simulink model "fxio_i2c_slave_rx_s32k11x"  (Simulink 9.0)
settings: Solver=FixedStepDiscrete  StartTime=0.0  StopTime=10.0  FixedStep=0.1  RelTol=1e-3
InitFcn:
  | mbd_s32k_consistency_checks(bdroot(gcs));
undefined symbols (not defined in the file): LQFP, thumb
libraries: mbd_s32k1xx_ec_toolbox x6, simulink x1
Description:
  | I2C Slave - to be used for FlexIO Master examples.
  | Note: FlexIO is limited to Master-only emulation for I2C - so LPI2C instance must be used for the Slave.
  | 
  | HW prerequisite:
  | - 2x S32K144 EVB (one running slave from this model), one master running fxio_master example.
  | - Connect:
  |     Master SDA - Slave SDA   : PTD0 (from this board) -  PTA2 (from master board)
  |     Master SCL - Slave SCL     : PTD1 (from this board) -  PTA3 (from master board)
  | 
  | Verification:
  | - for verification check FreeMASTER project for received data (on master button press, data should increment)
  | - LED should blink at every I2C STOP event
settings Model: Creator=nxf30742  LastModifiedBy=nxf35172
settings DataIOCC: ExternalInput=off  InitialState=off  SaveFormat=Dataset  SaveOutput=off  SignalLogging=off  SaveTime=off
settings OptimizationCC: DefaultParameterBehavior=Inlined  PassReuseOutputArgsAs=Individual arguments  LifeSpan=auto
settings DebuggingCC: UnderspecifiedInitializationDetection=Simplified  MergeDetectMultiDrivingBlocksExec=error  InheritedTsInSrcMsg=none  SingleTaskRateTransMsg=error  ParameterTunabilityLossMsg=error  UnconnectedInputMsg=error  UnconnectedOutputMsg=error  UnconnectedLineMsg=error  UnknownTsInhSupMsg=error  SFUnexpectedBacktrackingDiag=error  SFNoUnconditionalDefaultTransitionDiag=error  SFExecutionAtInitializationDiag=warning
settings HardwareCC: ProdLargestAtomicInteger=Long  ProdLargestAtomicFloat=Double  ProdIntDivRoundTo=Zero  ProdEndianess=LittleEndian  ProdHWDeviceType=ARM Compatible->ARM Cortex
settings ModelReferenceCC: PropagateSignalLabelsOutOfModel=on
settings SFSimCC: MATLABDynamicMemAlloc=off
settings RTWCC: SystemTargetFile=mbd_s32k.tlc  MakeCommand=mbd_s32k_make_rtw COPY_MDLREF_INCLUDES=0  TemplateMakefile=mbd_s32k.tmf  Description=Model Based Design Toolbox S32K14x Code Generation Target  GenerateReport=on  IncludeHyperlinkInReport=on  LaunchReport=on  GenerateTraceInfo=on  GenerateTraceReport=on  GenerateTraceReportSl=on  GenerateTraceReportSf=on  GenerateTraceReportEml=on
settings CodeAppCC: ForceParamTrailComments=on  IgnoreCustomStorageClasses=off  OperatorAnnotations=on  SimulinkDataObjDesc=on  SFDataObjDesc=on  InsertBlockDesc=on  StateflowObjectComments=off
settings STFCustomTargetCC: TargetLangStandard=C99 (ISO)  MultiwordLength=256  CombineOutputUpdateFcns=on  ERTCustomFileBanners=on  SupportContinuousTime=off  SupportNonInlinedSFcns=off  RemoveResetFunc=on  MATLABClassNameForMDSCustomization=Simulink.SoftwareTarget.ERTCustomization  GRTInterface=off  SystemTargetFile=mbd_s32k.tlc
settings ERTTargetCC: TargetLangStandard=C99 (ISO)  ParMdlRefBuildCompliant=off  CompOptLevelCompliant=off  ConcurrentExecutionCompliant=off  ModelStepFunctionPrototypeControlCompliant=off  CPPClassGenCompliant=off  UseToolchainInfoCompliant=off  InlinedParameterPlacement=NonHierarchical  ERTSrcFileBannerTemplate=mbd_ert_code_template.cgt  ERTHdrFileBannerTemplate=mbd_ert_code_template.cgt  ERTDataSrcFileTemplate=mbd_ert_code_template.cgt  ERTDataHdrFileTemplate=mbd_ert_code_template.cgt  ERTCustomFileTemplate=example_file_process.tlc
settings ConfigComp: CovMetricSettings=dwe  CovHtmlReporting=off  CovSaveCumulativeToWorkspaceVar=off  CovSaveSingleToWorkspaceVar=off  CovExternalEMLEnable=on

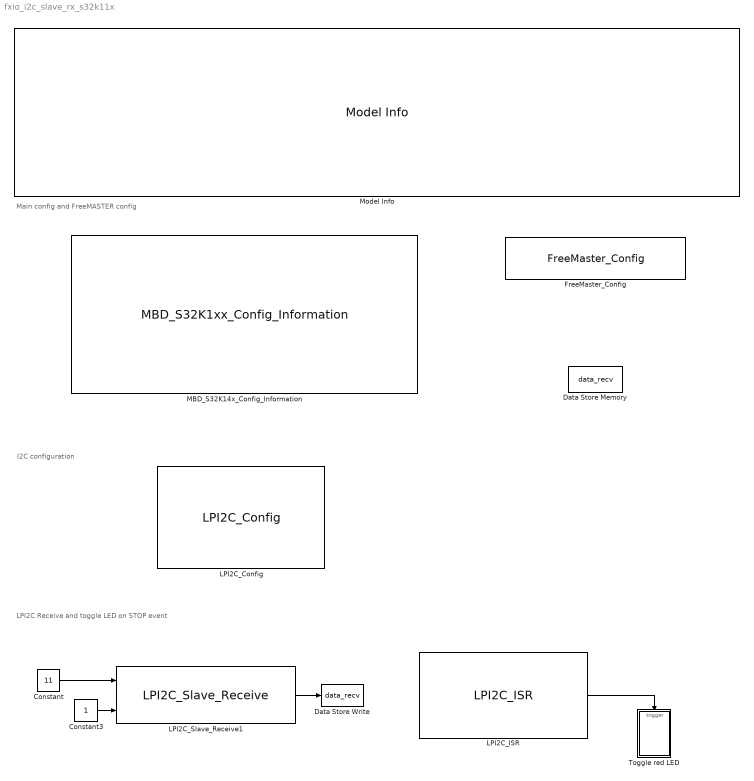
== system fxio_i2c_slave_rx_s32k11x ==
  note: Main config and FreeMASTER config
  note: LPI2C Receive and toggle LED on STOP event
  note: I2C configuration
  Constant : Constant  Value=11  OutDataTypeStr=uint16
  Constant3 : Constant  OutDataTypeStr=uint32
  Data Store Memory : DataStoreMemory  DataStoreName=data_recv  ReadBeforeWriteMsg=warning  WriteAfterWriteMsg=warning  WriteAfterReadMsg=warning  InitialValue=12  ShowAdditionalParam=off  OutDataTypeStr=uint8
  Data Store Write : DataStoreWrite  DataStoreName=data_recv
  FreeMaster_Config : mbd_s32k1xx_ec_toolbox/Utility Blocks/FreeMaster_Config  interface=LPUART0  baudrate=115200  rxd=PTB0: [LPUART0_RX | Receive]  txd=PTB1: [LPUART0_TX | Transmit]  mode=Short Interrupt  isr_prio=2  show_adv_opts=on  use_scope=on  max_scope_vars=8  use_recorder=on  max_rec_vars=8  rec_buff_size=1024  rec_timebase=0 seconds  comm_buffer_size_auto=on  comm_buffer_size=255  comm_rqueue_size_default=on  comm_rqueue_size=32
  LPI2C_Config : mbd_s32k1xx_ec_toolbox/Communication Blocks/I2C Blocks/LPI2C_Config  Priority=2  instance=0  mode=Slave  opmode=Standard (up to 100 kbit/s)  bdr=100000  addr=1  is10bitaddr=off  sda=PTA2: [LPI2C0_SDA | LPI2C Data I/O]  scl=PTA3: [LPI2C0_SCL | LPI2C Clock I/O]
  LPI2C_ISR : mbd_s32k1xx_ec_toolbox/Communication Blocks/I2C Blocks/LPI2C_ISR  instance=0  mode=Slave  rxreq=off  txreq=off  txempty=off  rxfull=off  stop=on  masterendtransfer=off  mastertx=off  masterrx=off  masterfifoerr=off  masterarblost=off  masternack=off
  LPI2C_Slave_Receive1 : mbd_s32k1xx_ec_toolbox/Communication Blocks/I2C Blocks/LPI2C_Slave_Receive  instance=0  xfermode=Non blocking  Timeout=300  is10bit=off
  MBD_S32K14x_Config_Information : mbd_s32k1xx_ec_toolbox/MBD_S32K1xx_Config_Information  Priority=1  mbdt_ver=0  disp_str=|  config_params=[]  mcu_target_name=S32K118  mcu_target_package=64-LQFP  mcu_target_sram_size=25KB  mcu_system_clock_freq=40  mcu_xtal_freq=External 40  mcu_steptick_timer=LPIT Channel 0  mcu_steptick_prio=0  ds_import_enable=on  target_compiler=GCC  target_memory=FLASH  gcc_target_compile_opts=-mcpu=cortex-m0plus -mthumb -O1 -g -gstrict-dwarf  gcc_target_assemble_opts=-mcpu=cortex-m0plus -mthumb -g  gcc_target_link_opts=-mcpu=cortex-m0plus -mthumb  gcc_target_default_lcf=on  gcc_target_user_lcf=S32K118_25_flash.ld  ghs_target_compile_opts=-mcpu=cortexm0plus -mthumb -fsoft -Ogeneral -Wundef -Wimplicit-int -Wshadow -Wtrigraphs --no_commons --gnu_asm -gnu99 -gdwarf-2 -G  ghs_target_assemble_opts=-mcpu=cortexm0plus -mthumb -fsoft --gnu_asm  ghs_target_link_opts=-mcpu=cortexm0plus -mthumb -fsoft  ghs_target_default_lcf=on  ghs_target_user_lcf=S32K118_25_flash.ld  iar_target_compile_opts=--thumb -Ol -e --debug --dlib_config normal  iar_target_assemble_opts=--thumb  iar_target_link_opts=--no_exceptions --vfe --inline  iar_target_default_lcf=on  iar_target_user_lcf=S32K118_25_flash.icf  pil_download_enable=off  rbl_download_enable=on  rbl_start_delay=5000000  rbl_download_interface=OpenSDA  rbl_restart_request=off  rbl_com_port=Custom  rbl_com_port_custom=COM1  pil_download_rate=57600  pil_opensda_drive=Custom  pil_opensda_drive_custom=D  pil_uart_instance=0  pil_uart_rx=PTB0: [LPUART0_RX | Receive]  pil_uart_tx=PTB1: [LPUART0_TX | Transmit]  FTM_PWM_PcrCheckEnDis=on  FTM_Input_Edge_Inputs_PcrCheckEnDis=on  FTM_Dual_Edge_Inputs_PcrCheckEnDis=on  FTM_Quadrature_Inputs_PcrCheckEnDis=on  FTM_Hall_Sensor_Inputs_PcrCheckEnDis=on  LPTMR_PcrCheckEnDis=on  PIT_PcrCheckEnDis=on  RTC_PcrCheckEnDis=on  FlexCAN_PcrCheckEnDis=on  LIN_PcrCheckEnDis=on  FlexIO_PcrCheckEnDis=on  LPI2C_PcrCheckEnDis=on  LPSPI_PcrCheckEnDis=on  LPUART_PcrCheckEnDis=on  CMP_PcrCheckEnDis=on  GPIO_OutputPcrCheckEnDis=on  GPIO_InputPcrCheckEnDis=on  SBC_PcrCheckEnDis=on  AMMCLIB_PcrCheckEnDis=on  FM_PcrCheckEnDis=on  Profile_PcrCheckEnDis=on  ConfigParams_PcrCheckEnDis=on  ModelRef_PcrCheckEnDis=on  PDB0_PcrCheckEnDis=on  CSEc_PcrCheckEnDis=on  eDMA_PcrCheckEnDis=on  ADC_PcrCheckEnDis=on  WDOG_PcrCheckEnDis=on
      | Target : S32K144-64KB_SRAM
      | Package : 100-pin
      | System clock : 80 MHz
      | XTAL clock : External 8 MHz
      | Compiler : GreenHills Multi
      | Target Type : FLASH
      | Download Code after build : off
      | Step Tick Interrupt Priority : 15
  Model Info : simulink/Model-Wide Utilities/Model Info  Frame=off  DisplayStringWithTags=|  HorizontalTextAlignment=Left  LeftAlignmentValue=0.02
      | Model Name: %<ModelName>
      | 
      | Description: %<Description>
  Toggle red LED : Subsystem
  wires:
  LPI2C_Slave_Receive1/1 -> Data Store Write/1
  Constant3/1 -> LPI2C_Slave_Receive1/2
  Constant/1 -> LPI2C_Slave_Receive1/1
  LPI2C_ISR/1 -> Toggle red LED/Trigger

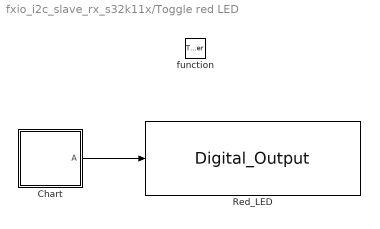
== system fxio_i2c_slave_rx_s32k11x/Toggle red LED ==
  function : TriggerPort  TriggerType=function-call  VariantControl=Variant
  Chart : Stateflow chart  TreatAsAtomicUnit=on
  Red_LED : mbd_s32k1xx_ec_toolbox/GPIO Blocks/Digital_Output  gpio_pin=PTD16: [PTD16 | Port D I/O]  init_val=Low  drive_strength=Low
  wires:
  Chart/1(" A") -> Red_LED/1

== stateflow chart Toggle red LED/Chart ==
  state A
  state A1
  (default) -> A
  A -> A1
  A1 -> A
  data: A output boolean [0..1]
